simulink model "Inv_Pend_HInf4"  (R2023b)
settings: Solver=VariableStepAuto  StartTime=0.0  StopTime=50  RelTol=1e-3
undefined symbols (not defined in the file): b, g, J, L, M, m
libraries: cstblocks x2
settings Model: Creator=DELL  LastModifiedBy=DELL

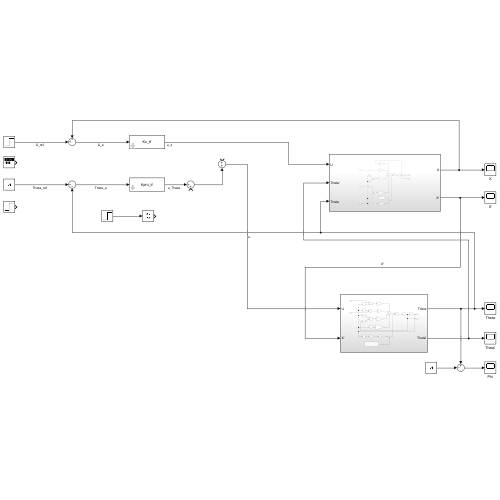
[thumbnail: Simulink's stored preview of the top-level diagram]
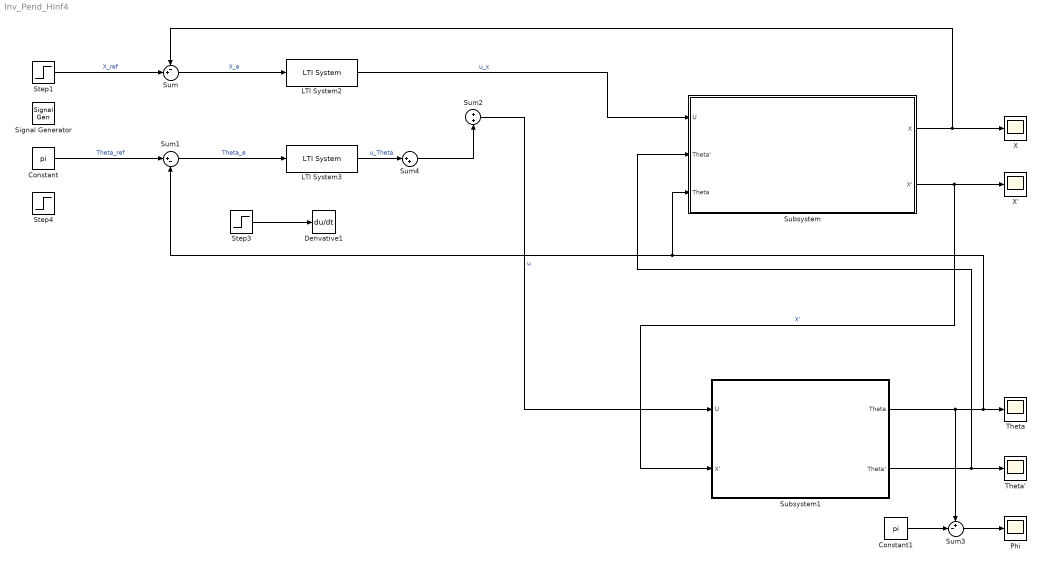
== system Inv_Pend_HInf4 ==
  Constant : Constant  Value=pi
  Constant1 : Constant  Value=pi
  Derivative1 : Derivative
  LTI System2 : cstblocks/LTI System  sys=Kx_tf  IC=[]  PadeOrder=0
  LTI System3 : cstblocks/LTI System  sys=Kphi_tf  IC=[]  PadeOrder=0
  Phi : Scope
  Signal Generator : SignalGenerator  Units=rad/sec
  Step1 : Step  After=3  SampleTime=0
  Step3 : Step  After=50  SampleTime=0
  Step4 : Step  SampleTime=0
  Subsystem : Subsystem
  Subsystem1 : Subsystem
  Sum : Sum  Inputs=-+|
  Sum1 : Sum  Inputs=|+-
  Sum2 : Sum  Inputs=+|+
  Sum3 : Sum  Inputs=+-|
  Sum4 : Sum  Inputs=|++
  Theta : Scope
  Theta' : Scope
  X : Scope
  X' : Scope
  wires:
  LTI System3/1 -> Sum4/1  "u_Theta"
  Sum/1 -> LTI System2/1  "X_e"
  Sum1/1 -> LTI System3/1  "Theta_e"
  Sum4/1 -> Sum2/2
  Step3/1 -> Derivative1/1
  Constant/1 -> Sum1/1  "Theta_ref"
  Step1/1 -> Sum/2  "X_ref"
  Subsystem1/2(Theta') -> Theta'/1, Subsystem/2(Theta')
  Subsystem/2(X') -> X'/1, Subsystem1/2(X')  "X'"
  Subsystem1/1(Theta) -> Sum3/1, Sum1/2, Subsystem/3(Theta), Theta/1
  Sum2/1 -> Subsystem1/1(U)  "u"
  Sum3/1 -> Phi/1
  Constant1/1 -> Sum3/2
  Subsystem/1(X) -> Sum/1, X/1
  LTI System2/1 -> Subsystem/1(U)  "u_x"

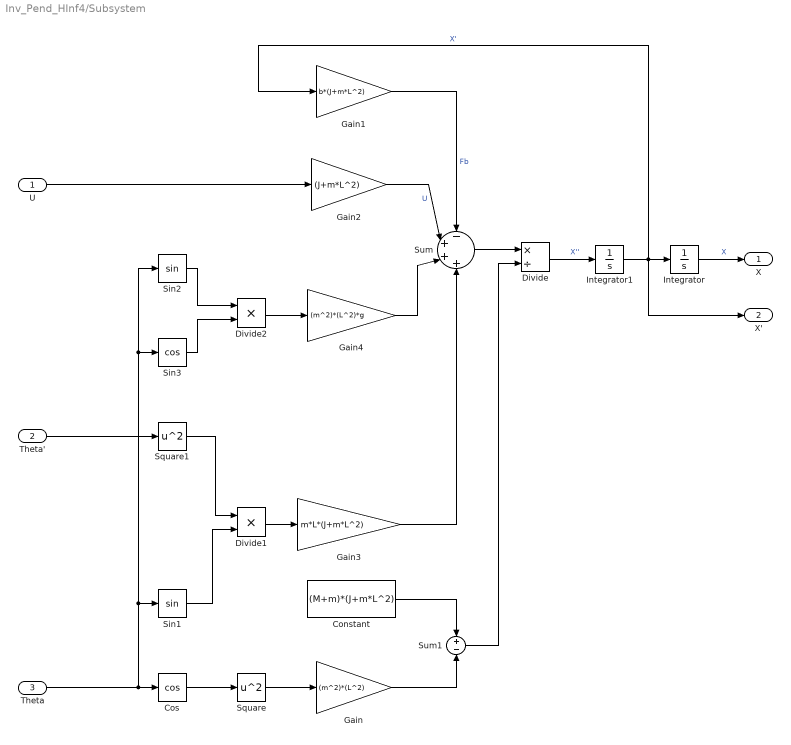
== system Inv_Pend_HInf4/Subsystem ==
  U : Inport
  Theta' : Inport  Port=2
  Theta : Inport  Port=3
  Constant : Constant  Value=(M+m)*(J+m*L^2)
  Cos : Trigonometry  Operator=cos
  Divide : Product  Inputs=*/
  Divide1 : Product  Inputs=**
  Divide2 : Product  Inputs=**
  Gain : Gain  Gain=(m^2)*(L^2)
  Gain1 : Gain  Gain=b*(J+m*L^2)
  Gain2 : Gain  Gain=(J+m*L^2)
  Gain3 : Gain  Gain=m*L*(J+m*L^2)
  Gain4 : Gain  Gain=(m^2)*(L^2)*g
  Integrator : Integrator
  Integrator1 : Integrator
  Sin1 : Trigonometry
  Sin2 : Trigonometry
  Sin3 : Trigonometry  Operator=cos
  Square : Math  Operator=square
  Square1 : Math  Operator=square
  Sum : Sum  Inputs=-+++
  Sum1 : Sum  Inputs=+|-
  X : Outport
  X' : Outport  Port=2
  wires:
  Square/1 -> Gain/1
  Square1/1 -> Divide1/1
  Theta/1 -> Sin2/1, Sin3/1, Sin1/1, Cos/1
  Integrator1/1 -> X'/1, Gain1/1, Integrator/1  "X'"
  Constant/1 -> Sum1/1
  Divide/1 -> Integrator1/1  "X''"
  Sin1/1 -> Divide1/2
  Integrator/1 -> X/1  "X"
  Gain1/1 -> Sum/1  "Fb"
  Cos/1 -> Square/1
  Sum/1 -> Divide/1
  Divide2/1 -> Gain4/1
  Gain/1 -> Sum1/2
  Sin3/1 -> Divide2/2
  U/1 -> Gain2/1
  Sum1/1 -> Divide/2
  Sin2/1 -> Divide2/1
  Theta'/1 -> Square1/1
  Gain3/1 -> Sum/4
  Divide1/1 -> Gain3/1
  Gain4/1 -> Sum/3
  Gain2/1 -> Sum/2  "U"

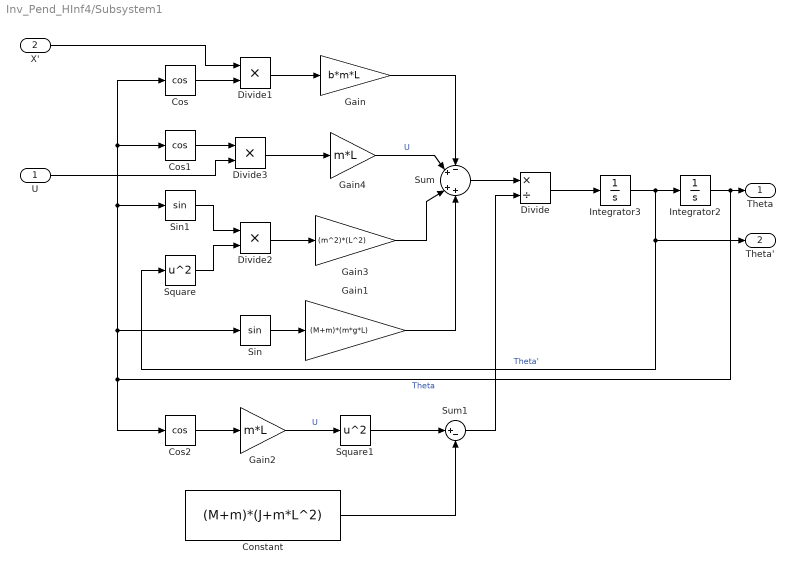
== system Inv_Pend_HInf4/Subsystem1 ==
  U : Inport
  X' : Inport  Port=2
  Constant : Constant  Value=(M+m)*(J+m*L^2)
  Cos : Trigonometry  Operator=cos
  Cos1 : Trigonometry  Operator=cos
  Cos2 : Trigonometry  Operator=cos
  Divide : Product  Inputs=*/
  Divide1 : Product  Inputs=**
  Divide2 : Product  Inputs=**
  Divide3 : Product  Inputs=**
  Gain : Gain  Gain=b*m*L
  Gain1 : Gain  Gain=(M+m)*(m*g*L)
  Gain2 : Gain  Gain=m*L
  Gain3 : Gain  Gain=(m^2)*(L^2)
  Gain4 : Gain  Gain=m*L
  Integrator2 : Integrator
  Integrator3 : Integrator
  Sin : Trigonometry
  Sin1 : Trigonometry
  Square : Math  Operator=square
  Square1 : Math  Operator=square
  Sum : Sum  Inputs=-+|++
  Sum1 : Sum  Inputs=|+-
  Theta : Outport
  Theta' : Outport  Port=2
  wires:
  Gain4/1 -> Sum/2  "U"
  Gain/1 -> Sum/1
  Gain3/1 -> Sum/3
  Square/1 -> Divide2/2
  Divide1/1 -> Gain/1
  Cos1/1 -> Divide3/1
  Sin/1 -> Gain1/1
  Divide2/1 -> Gain3/1
  Sin1/1 -> Divide2/1
  Divide3/1 -> Gain4/1
  Sum/1 -> Divide/1
  Divide/1 -> Integrator3/1
  Cos/1 -> Divide1/2
  Gain1/1 -> Sum/4
  Integrator2/1 -> Cos2/1, Sin/1, Cos/1, Cos1/1, Sin1/1, Theta/1  "Theta"
  U/1 -> Divide3/2
  X'/1 -> Divide1/1
  Integrator3/1 -> Theta'/1, Square/1, Integrator2/1  "Theta'"
  Gain2/1 -> Square1/1  "U"
  Cos2/1 -> Gain2/1
  Square1/1 -> Sum1/1
  Sum1/1 -> Divide/2
  Constant/1 -> Sum1/2
